simulink model "dev_sim_lqg"  (R2019b)
settings: Solver=VariableStepAuto  StartTime=0.0  StopTime=200.0  RelTol=1e-3
values from neighbouring files (symbols this model uses):
  A_0 = eval(A_0)    [modelo.m]    (also in modelo_var.m; parametros.mat = [0 -3.26931291643 0 0.71460251427 0 0 0 0 1 -0.0325743287495)
  B_0 = eval(B_0)    [modelo.m]    (also in modelo_var.m; parametros.mat = [0 0 0 0 0 0 1190.47619048 0 0 0 0 0 ... (16 elements, 8x2)])
  C_0 = eval(C_0)    [modelo.m]    (also in modelo_var.m; parametros.mat = [1 0 0 0 0 1 0 0 0 0 0 0 ... (16 elements, 2x8)])
  D_0 = eval(D_0)    [modelo.m]    (also in modelo_var.m; parametros.mat = [0  0; 0  0])
  L = Ec-Ep    [modelo.m]    (also in modelo_var.m)
  u0 = [u_p_0;u_t_0]    [modelo.m]    (also in modelo_var.m; parametros.mat = [11.9668031953 -0.0853053139382])
  x0 = [phi_0; d_phi_0; theta_0; d_theta_0; w_p_0; w_t_0; i_p_0; i_t_0]    [modelo.m]    (also in modelo_var.m; parametros.mat = [0.0001 0 0 0 65.3284351132 -0.694344279837 0.788144659543 -)
  xinit = x0 - [0.1; 0.1; 0.1; 0.1; 0.1; 0.1; 0.1; 0.1]    [modelo_var.m]
undefined symbols (not defined in the file or in its folder): K
settings Model: Creator=tronc  LastModifiedBy=tronc

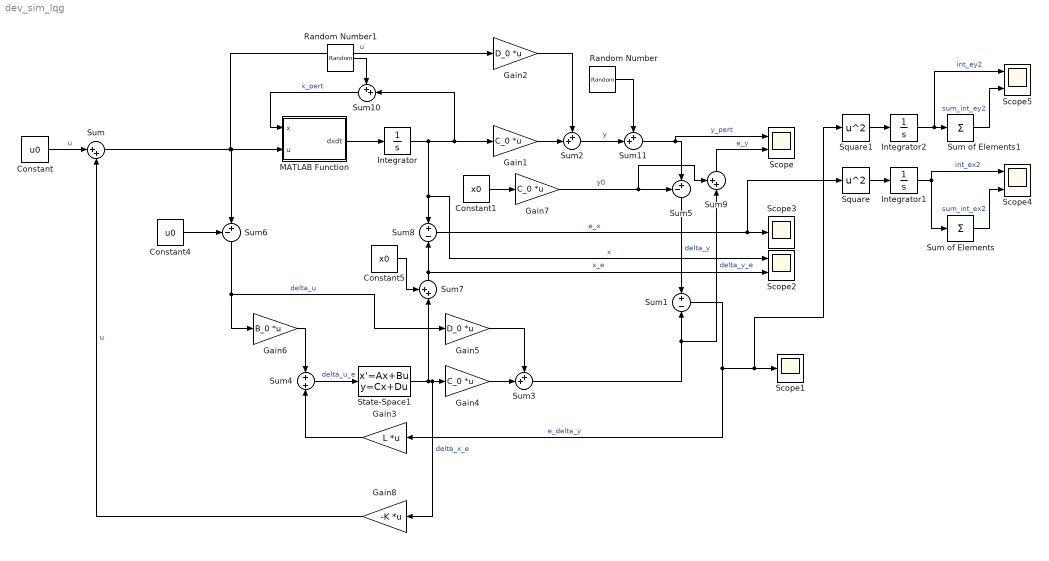
== system dev_sim_lqg ==
  Constant : Constant  Value=u0
  Constant1 : Constant  Value=x0
  Constant4 : Constant  Value=u0
  Constant5 : Constant  Value=x0
  Gain1 : Gain  Gain=C_0  Multiplication=Matrix(K*u)
  Gain2 : Gain  Gain=D_0  Multiplication=Matrix(K*u)
  Gain3 : Gain  Gain=L  Multiplication=Matrix(K*u)
  Gain4 : Gain  Gain=C_0  Multiplication=Matrix(K*u)
  Gain5 : Gain  Gain=D_0  Multiplication=Matrix(K*u)
  Gain6 : Gain  Gain=B_0  Multiplication=Matrix(K*u)
  Gain7 : Gain  Gain=C_0  Multiplication=Matrix(K*u)
  Gain8 : Gain  Gain=-K  Multiplication=Matrix(K*u)
  Integrator : Integrator  InitialCondition=xinit
  Integrator1 : Integrator
  Integrator2 : Integrator
  MATLAB Function : MATLAB Function  TreatAsAtomicUnit=on
  Random Number : RandomNumber  Variance=0.0001  SampleTime=0.1
  Random Number1 : RandomNumber  Variance=0.0001  SampleTime=0.1
  Scope{,2,4..5} (4 alike) : Scope  NumInputPorts=2
  Scope1 : Scope
  Scope3 : Scope
  Square : Math  Operator=square  SignedPower=off  SaturateOnIntegerOverflow=on
  Square1 : Math  Operator=square  SignedPower=off  SaturateOnIntegerOverflow=on
  State-Space1 : StateSpace  A=A_0  B=eye(8)  C=eye(8)  D=zeros(8)  InitialCondition=[0.1 0.1 0.1 0.1 0.1 0.1 0.1 0.1]
  Sum : Sum  Inputs=|++
  Sum of Elements : Sum  Inputs=+
  Sum of Elements1 : Sum  Inputs=+
  Sum1 : Sum  Inputs=+|-
  Sum{2..3,7,9..11} (6 alike) : Sum  Inputs=++|
  Sum4 : Sum  Inputs=+|+
  Sum5 : Sum  Inputs=-+|
  Sum6 : Sum  Inputs=-+|
  Sum8 : Sum  Inputs=+-
  wires:
  MATLAB Function/1(dxdt) -> Integrator/1
  Integrator/1 -> Scope2/1, Sum8/1, Sum10/2, Gain1/1  "x"
  Gain1/1 -> Sum2/2
  Gain2/1 -> Sum2/1
  Sum/1 -> Sum6/2, MATLAB Function/2(u), Gain2/1  "u"
  Sum4/1 -> State-Space1/1  "delta_u_e"
  State-Space1/1 -> Sum7/2, Gain8/1, Gain4/1  "delta_x_e"
  Gain3/1 -> Sum4/2
  Sum1/1 -> Gain3/1, Square1/1, Scope1/1  "e_delta_y"
  Gain6/1 -> Sum4/1
  Sum3/1 -> Sum9/2, Sum1/2  "delta_y_e"
  Gain4/1 -> Sum3/2
  Gain5/1 -> Sum3/1
  Sum11/1 -> Scope/1, Sum5/2  "y_pert"
  Sum5/1 -> Sum1/1  "delta_y"
  Constant1/1 -> Gain7/1
  Gain7/1 -> Sum9/1, Sum5/1  "y0"
  Sum6/1 -> Gain5/1, Gain6/1  "delta_u"
  Constant4/1 -> Sum6/1
  Constant5/1 -> Sum7/1
  Sum7/1 -> Sum8/2, Scope2/2  "x_e"
  Sum8/1 -> Square/1, Scope3/1  "e_x"
  Sum10/1 -> MATLAB Function/1(x)  "x_pert"
  Sum2/1 -> Sum11/2  "y"
  Random Number/1 -> Sum11/1
  Random Number1/1 -> Sum10/1
  Square/1 -> Integrator1/1
  Integrator1/1 -> Sum of Elements/1, Scope4/1  "int_ex2"
  Sum of Elements/1 -> Scope4/2  "sum_int_ex2"
  Sum9/1 -> Scope/2  "e_y"
  Square1/1 -> Integrator2/1
  Sum of Elements1/1 -> Scope5/2  "sum_int_ey2"
  Integrator2/1 -> Scope5/1, Sum of Elements1/1  "int_ey2"
  Constant/1 -> Sum/1  "u"
  Gain8/1 -> Sum/2  "u"

== matlab function dev_sim_lqg/MATLAB Function ==
  data: x input; u input; dxdt output
function dxdt = fcn(x,u)
phi = x(1);d_phi = x(2);theta = x(3);d_theta = x(4);w_p = x(5); w_t = x(6); i_p = x(7); i_t = x(8);
u_p = u(1); u_t = u(2);
dxdt = [d_phi;
(((2231553*cos(phi)^2)/4000000 + 6271303914229987/36028797018963968)*((3*d_phi)/250 - (27043227*cos(phi))/20000000 + (3022461*sin(phi))/2500000 + (1256252657407189*d_theta^2*sin(2*phi))/9007199254740992 + (2921964261275593*w_p*abs(w_p))/9223372036854775808))/((1566754414544131*cos(phi)*sin(phi))/9223372036854775808 - (1850992331451507*cos(phi)^2)/9007199254740992 + (3504602316272157*sin(phi)^2)/36893488147419103232 - 4621850957490069/72057594037927936) - (((1027*cos(phi))/25000 + (9189*sin(phi))/200000)*((6466506135038883*w_t*abs(w_t))/368934881474191032320 - (9*d_theta)/5000 + (9*d_phi^2*((9189*cos(phi))/200000 - (1027*sin(phi))/25000))/200 + (1507503188888627*d_phi*d_theta*sin(2*phi))/18014398509481984 + (7304910653188983*w_p*abs(w_p)*sin(phi))/368934881474191032320))/((1566754414544131*cos(phi)*sin(phi))/9223372036854775808 - (1850992331451507*cos(phi)^2)/9007199254740992 + (3504602316272157*sin(phi)^2)/36893488147419103232 - 4621850957490069/72057594037927936);
d_theta;
(((1027*cos(phi))/25000 + (9189*sin(phi))/200000)*((9*d_phi)/2500 - (81129681*cos(phi))/200000000 + (9067383*sin(phi))/25000000 + (1507503188888627*d_theta^2*sin(2*phi))/36028797018963968 + (438294639191339*w_p*abs(w_p))/4611686018427387904))/((1566754414544131*cos(phi)*sin(phi))/9223372036854775808 - (1850992331451507*cos(phi)^2)/9007199254740992 + (3504602316272157*sin(phi)^2)/36893488147419103232 - 4621850957490069/72057594037927936) - ((3177141253833869*w_t*abs(w_t))/73786976294838206464 - (4978621639436999*d_theta)/1125899906842624000 + (4978621639436999*d_phi^2*((9189*cos(phi))/200000 - (1027*sin(phi))/25000))/45035996273704960 + (7406705370233703*d_phi*d_theta*sin(2*phi))/36028797018963968 + (7178136850767151*w_p*abs(w_p)*sin(phi))/147573952589676412928)/((1566754414544131*cos(phi)*sin(phi))/9223372036854775808 - (1850992331451507*cos(phi)^2)/9007199254740992 + (3504602316272157*sin(phi)^2)/36893488147419103232 - 4621850957490069/72057594037927936);
(74600*i_p)/1083 - (300*w_p)/361;
(1492000*i_t)/10609 - (8000*w_t)/10609;
(25000*u_p)/21 - (75000*i_p)/7 - (1865*w_p)/21;
(25000*u_t)/21 - (75000*i_t)/7 - (1865*w_t)/21;
];
